simulink model "Lichtsteuerung_leer"  (R2025b)
settings: Solver=FixedStepDiscrete  StartTime=0  StopTime=50  FixedStep=0.01  RelTol=1e-3  EnableMultiTasking=on
settings Model: RequirementInfo={} %GIDa_e5b38421_296d_4fa5_bc87_66157657de61  ExtModeTrigMode=oneshot  Creator=martin  LastModifiedBy=danieltchoudovski
settings SolverCC: AlgebraicLoopSolver=TrustRegion
settings DataIOCC: SaveFormat=Array  SignalLoggingSaveFormat=ModelDataLogs  SaveOutput=off  SaveTime=off  ReturnWorkspaceOutputs=off  SignalLoggingName=sigsOut
settings OptimizationCC: BlockReduction=off  BooleanDataType=off  OptimizeBlockIOStorage=off  BufferReuse=off  GlobalBufferReuse=off  ExpressionFolding=off  ExpressionDepthLimit=2147483647.0  LocalBlockOutputs=off  InitFltsAndDblsToZero=on  LifeSpan=inf  OptimizeDataStoreBuffers=off  BusAssignmentInplaceUpdate=off
settings DebuggingCC: SaveWithParameterizedLinksMsg=none  UnderspecifiedInitializationDetection=Classic  MergeDetectMultiDrivingBlocksExec=none  SignalResolutionControl=TryResolveAllWithWarning  MultiTaskDSMMsg=warning  MultiTaskCondExecSysMsg=none  FcnCallInpInsideContextMsg=warning  UnconnectedInputMsg=warning  UnconnectedOutputMsg=warning  UnconnectedLineMsg=warning  StateNameClashWarn=warning  SFUnexpectedBacktrackingDiag=warning  SFNoUnconditionalDefaultTransitionDiag=warning  SFExecutionAtInitializationDiag=none  ArithmeticOperatorsInVariantConditions=warning
settings HardwareCC: ProdBitPerPointer=32.0  ProdBitPerSizeT=32.0  ProdBitPerPtrDiffT=32.0  ProdLargestAtomicFloat=None  ProdIntDivRoundTo=Undefined  ProdEndianess=Unspecified  ProdWordSize=32.0  ProdHWDeviceType=32-bit Generic  TargetBitPerLong=64.0  TargetBitPerPointer=64.0  TargetBitPerSizeT=64.0  TargetBitPerPtrDiffT=64.0  TargetLongLongMode=on  TargetIntDivRoundTo=Zero  TargetEndianess=LittleEndian  TargetWordSize=64.0  TargetHWDeviceType=MATLAB Host  ProdEqTarget=off
settings ModelReferenceCC: EnableRefExpFcnMdlSchedulingChecks=on  PropagateSignalLabelsOutOfModel=off
settings SFSimCC: SimUseLocalCustomCode=off  SimParseCustomCode=off  CustomCodeUndefinedFunction=UseInterfaceOnly
settings RTWCC: GenerateReport=on  RTWUseLocalCustomCode=off  GPUComputeCapability=3.5
settings CodeAppCC: StateflowObjectComments=on
settings GRTTargetCC: ExtMode=on  TargetLangStandard=C89/C90 (ANSI)  CombineOutputUpdateFcns=off  GRTInterface=on
settings ConfigComp: CovMetricSettings=dw  CovSaveCumulativeToWorkspaceVar=on  CovSaveSingleToWorkspaceVar=on  CovExternalEMLEnable=off

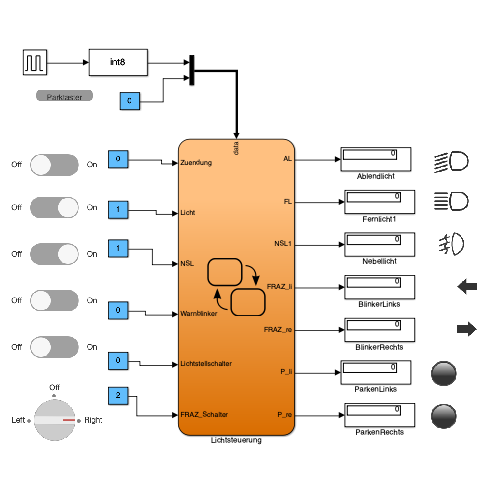
[thumbnail: Simulink's stored preview of the top-level diagram]
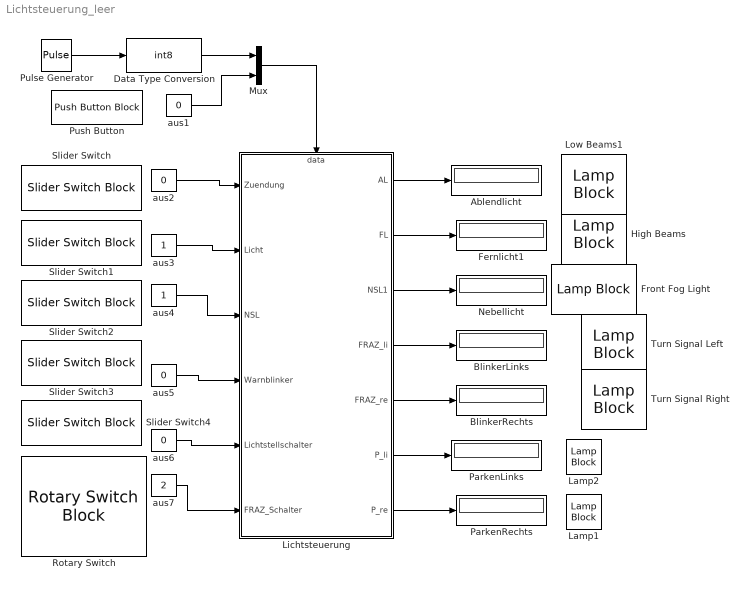
== system Lichtsteuerung_leer ==
  Ablendlicht : Display
  BlinkerLinks : Display
  BlinkerRechts : Display
  Data Type Conversion : DataTypeConversion  OutDataTypeStr=int8  SaturateOnIntegerOverflow=off  RndMeth=Floor
  Fernlicht1 : Display
  Front Fog Light : LampBlock  LabelPosition=Hide  DefaultColor=[192.0, 192.0, 192.0]  Icon=FrontFogLight
  High Beams : LampBlock  LabelPosition=Hide  DefaultColor=[192.0, 192.0, 192.0]  Icon=HighBeams
  Lamp1 : LampBlock  LabelPosition=Hide  DefaultColor=[0.0, 0.0, 0.0]
  Lamp2 : LampBlock  LabelPosition=Hide  DefaultColor=[192.0, 192.0, 192.0]
  Lichtsteuerung : Stateflow chart  TreatAsAtomicUnit=on
      settings: PortSchema="{\"entries\":[{\"content\":{\"sides\":[{\"content\":{\"connectorIds\":[\"In5\",\"In2\",\"In3\",\"In4\",\"In6\",\"In7\"]},\"type\":\"ConnectorPlacement.EquallySpacedRectSide\",\"uuid\":\"f0ab4642-4e7a-4609-a7e9-6d2d3d58973a\"},{\"content\":{\"connectorIds\":[\"Out1\",\"Out2\",\"Out3\",\"Out4\",\"Out5\",\"Out6\",\"Out7\"],\"side\":\"RIGHT\"},\"type\":\"ConnectorPlacement.EquallySpacedRectSide\",\"uuid\":\"dceffa1b-49b7-452e-95ae-2b305586e5f6\"},{\"content\":{\"connectorIds\":[\"In1\"],\"side\":\"TOP\"},\"type\":\"ConnectorPlacement.EquallySpacedRectSide\",\"uuid\":\"ffbb170c-e657-4448-923f-e11daef6f64e\"}]},\"type\":\"ConnectorPlacement.EquallySpacedConnector\",\"uuid\":\"6e0992a5-cb09-4143-8eda-0609fad98602\"}],\"packageUris\":[\"http://schema.mathworks.com/mf0/Connector/R2020b\"],\"version\":\"1.0\"}"
  Low Beams1 : LampBlock  LabelPosition=Hide  DefaultColor=[192.0, 192.0, 192.0]  Icon=LowBeams
  Mux : Mux  Inputs=2
  Nebellicht : Display
  ParkenLinks : Display
  ParkenRechts : Display
  Pulse Generator : DiscretePulseGenerator  PulseType=Time based  Period=0.02  PulseWidth=50
  Push Button : PushButtonBlock  ButtonText=Parktaster  IconOnColor=[0.0, 0.39215686274509803, 0.0]  IconOffColor=[0.0, 1.0, 0.0]  OffValue=0.000000
  Rotary Switch : RotarySwitchBlock  LabelPosition=Hide
  Slider Switch{,1..4} (5 alike) : SliderSwitchBlock  LabelPosition=Hide
  Turn Signal Left : LampBlock  LabelPosition=Hide  DefaultColor=[192.0, 192.0, 192.0]  Icon=TurnSignalLeft
  Turn Signal Right : LampBlock  LabelPosition=Hide  DefaultColor=[192.0, 192.0, 192.0]  Icon=TurnSignalRight
  aus{1..2,5..6} (4 alike) : Constant  Value=0  OutDataTypeStr=int8
  aus3 : Constant  OutDataTypeStr=int8
  aus4 : Constant  OutDataTypeStr=int8
  aus7 : Constant  Value=2  OutDataTypeStr=int8
  wires:
  Mux/1 -> Lichtsteuerung/1(data)
  Lichtsteuerung/2(FL) -> Fernlicht1/1
  Lichtsteuerung/4(FRAZ_li) -> BlinkerLinks/1
  Lichtsteuerung/5(FRAZ_re) -> BlinkerRechts/1
  Lichtsteuerung/6(P_li) -> ParkenLinks/1
  Lichtsteuerung/1(AL) -> Ablendlicht/1
  Lichtsteuerung/3(NSL1) -> Nebellicht/1
  Lichtsteuerung/7(P_re) -> ParkenRechts/1
  aus4/1 -> Lichtsteuerung/3(NSL)
  aus5/1 -> Lichtsteuerung/4(Warnblinker)
  aus7/1 -> Lichtsteuerung/7(FRAZ_Schalter)
  aus2/1 -> Lichtsteuerung/5(Zuendung)
  aus6/1 -> Lichtsteuerung/6(Lichtstellschalter)
  aus3/1 -> Lichtsteuerung/2(Licht)
  Pulse Generator/1 -> Data Type Conversion/1
  Data Type Conversion/1 -> Mux/1
  aus1/1 -> Mux/2

== stateflow chart Lichtsteuerung_leer/Lichtsteuerung ==
  settings: executeAtInitialization=1  description=Steuerung für einen Gebläse mit Heizung
  state Zuendung [parallel]
    settings: executionOrder=2
    state Zuendung_aus
      en:
      AL=0;
      FL=0;
      NSL1=0;
      FRAZ_li_active=0;
      FRAZ_re_active=0;
      state Parklicht_inactive
        en:
        P_li=0;
        P_re=0;
      state Parklicht_active
        state Parklicht_aus
          en:
          P_li=0;
          P_re=0;
        state Parklicht_re
          en:
          P_re=1;
          exit:
          P_re=0;
        state Parklicht_li
          en:
          P_li=1;
          exit:
          P_li=0;
        (default) -> Parklicht_aus
        Parklicht_re -> Parklicht_aus : [FRAZ_Schalter==0]
        Parklicht_aus -> Parklicht_re [order 2] : [FRAZ_Schalter==2]
        Parklicht_aus -> Parklicht_li [order 1] : [FRAZ_Schalter==1]
        Parklicht_li -> Parklicht_aus : [FRAZ_Schalter==0]
      (default) -> Parklicht_inactive
      Parklicht_inactive -> Parklicht_active : [rising(data[1])]
      Parklicht_active -> Parklicht_inactive : [rising(data[1])]
    state Zuendung_an
      en:
      P_li=0;
      P_re=0;
      state Licht [parallel]
        settings: executionOrder=1
        state Licht_Aus
          en:
          AL = 0;
          FL = 0;
        state Licht_An
          state AL
            en:
            AL = 1;
            FL = 0;
          state NSL
            en:
            NSL1 = 1;
          state FL
            en:
            NSL1=0;
            AL = 0;
            FL = 1;
          (default) -> AL
          NSL -> AL [order 1] : [NSL == 0]
          AL -> NSL [order 2] : [NSL==1]
          FL -> AL : [Lichtstellschalter == 0]
          AL -> FL [order 1] : [Lichtstellschalter == 1]
          NSL -> FL [order 2] : [Lichtstellschalter==1]
        (default) -> Licht_Aus
        Licht_Aus -> Licht_An : [Licht == 1]
        Licht_An -> Licht_Aus : [Licht == 0]
      state FRAZ [parallel]
        settings: executionOrder=2
        state FRAZ_Aus
          en:
          FRAZ_li_active = 0;
          FRAZ_re_active = 0;
        state FRAZ_Re
          en:
          FRAZ_re_active=1;
          exit:
          FRAZ_re=0;
        state FRAZ_Li
          en:
          FRAZ_li_active=1;
          exit:
          FRAZ_li=0;
        (default) -> FRAZ_Aus
        FRAZ_Aus -> FRAZ_Li [order 1] : [FRAZ_Schalter == 1]
        FRAZ_Aus -> FRAZ_Re [order 2] : [FRAZ_Schalter == 2]
        FRAZ_Re -> FRAZ_Aus [order 1] : [FRAZ_Schalter == 0]
        FRAZ_Li -> FRAZ_Aus [order 1] : [FRAZ_Schalter == 0]
        FRAZ_Li -> FRAZ_Aus [order 2] : e_WB
        FRAZ_Re -> FRAZ_Aus [order 2] : e_WB
    (default) -> Zuendung_aus
    Zuendung_aus -> Zuendung_an : [Zuendung==1]
    Zuendung_an -> Zuendung_aus : [Zuendung==0]
  state FRAZ_li [parallel]
    settings: executionOrder=3
    state on_on
      en:
      FRAZ_li=1;
    state off
      en:
      FRAZ_li=0;
    state on_off
      en:
      FRAZ_li=0;
    (default) -> FRAZ_li.on_on [order 2] : e_WB
    (default) -> FRAZ_li.off [order 1]
    FRAZ_li.off -> FRAZ_li.on_on : [FRAZ_li_active==1]
    FRAZ_li.on_on -> FRAZ_li.off [order 1] : [FRAZ_li_active == 0]
    FRAZ_li.on_off -> FRAZ_li.on_on : after(0.5,sec)
    FRAZ_li.on_on -> FRAZ_li.on_off [order 2] : after(0.5,sec)
  state FRAZ_re [parallel]
    settings: executionOrder=4
    state on_on
      en:
      FRAZ_re=1;
    state off
      en:
      FRAZ_re=0;
    state on_off
      en:
      FRAZ_re=0;
    (default) -> FRAZ_re.on_on [order 2] : e_WB
    (default) -> FRAZ_re.off [order 1]
    FRAZ_re.off -> FRAZ_re.on_on : [FRAZ_re_active==1]
    FRAZ_re.on_on -> FRAZ_re.off [order 1] : [FRAZ_re_active == 0]
    FRAZ_re.on_off -> FRAZ_re.on_on : after(0.5,sec)
    FRAZ_re.on_on -> FRAZ_re.on_off [order 2] : after(0.5,sec)
  state Warnblinker [parallel]
    settings: executionOrder=1
    state Warnblinker_an
      en:
      send(e_WB);
      FRAZ_li_active=1;
      FRAZ_re_active=1;
    state Warnblinker_aus
      en:
      send(e_WB);
    (default) -> Warnblinker_aus
    Warnblinker_an -> Warnblinker_aus : [Warnblinker==0]
    Warnblinker_aus -> Warnblinker_an : [Warnblinker==1]
  data: data input; AL output double; FL output double; NSL1 output; Licht input; NSL input; Warnblinker input; Zuendung input; Lichtstellschalter input; FRAZ_Schalter input; FRAZ_li output double; FRAZ_re output double; P_li output double; P_re output double; FRAZ_li_active local int8; FRAZ_re_active local int8
  events: e_WB local FUNCTION_CALL_EVENT
